simulink model "rev0BB"  (R2017b)
settings: Solver=FixedStepDiscrete  StartTime=0  StopTime=(((preLen+100+dataLenSymbols)*1+pad_first*3)*basePer)  RelTol=1e-3
values from neighbouring files (symbols this model uses):
  ack_stf_len_symbols = length(x_ACK_STF)    [rev0BB_setup.m]
  agc_delay_lag = 32    [rev0BB_setup.m]
  agc_detector_coef = ones(1,agc_detector_taps)./agc_detector_taps    [rev0BB_setup.m]
  agc_on = true    [rev0BB_startup.m]
  agc_sat_low = -agcSaturation    (= -12)    [rev0BB_setup.m]
  agc_sat_up = agcSaturation    (= 12)    [rev0BB_setup.m]
  agcDesired = 0    [rev0BB_setup.m]
  agcExpDomain = agcSaturation    (= 12)    [rev0BB_setup.m]
  agcExpResolution = 2^-5    (= 0.03125)    [rev0BB_setup.m]
  agcPwrAvgNum = 128    [rev0BB_setup.m]
  agcSaturation = 12    [rev0BB_setup.m]
  agcSettleThresh = 0.65    [rev0BB_setup.m]
  agcStep = 2^-8    (= 0.00390625)    [rev0BB_setup.m]
  atanDomain = 5    [rev0BB_setup.m]
  atanDomainTiming = 256    [rev0BB_setup.m]
  atanResolution = 2^-9    (= 0.001953125)    [rev0BB_setup.m]
  atanResolutionTiming = 2^-5    (= 0.03125)    [rev0BB_setup.m]
  averaging_num = ones(1, averaging_samples)    [rev0BB_setup.m]
  averaging_samples = 128    [rev0BB_setup.m]
  awgnSeed = abs(dBSnrRange(dBSnrInd)*1000+trial+10000000)    [plotBer.m]    (also in rev0BB_startup.m = 67)
  basePer = 1/baseFreq    (= 5e-08)    [rev0BB_setup.m]
  bitsPerSymbolHeader = log2(radixHeader)    [rev0BB_setup.m]
  bitsPerSymbolMax = log2(radixMax)    [rev0BB_setup.m]
  cal_sig_i_mult = 1.0    (= 1)    [rev0BB_startup.m]
  cal_sig_i_offset = 0.0    (= 0)    [rev0BB_startup.m]
  cal_sig_q_mult = 1.0    (= 1)    [rev0BB_startup.m]
  cal_sig_q_offset = 0.0    (= 0)    [rev0BB_startup.m]
  cefEarlyWarning = 256    [rev0BB_setup.m]
  cefLen = length(x_CEF)    [rev0BB_setup.m]
  channelFIR = zeros(1, round(maxSampleDelay)+1)    [rev0BB_startup.m]
  coarseCFOAdaptDelay = 1    [rev0BB_setup.m]
  cr_i = 0.020    (= 0.02)    [rev0BB_setup.m]
  cr_i_preamp = 2^-9    (= 0.001953125)    [rev0BB_setup.m]
  cr_int1_sat_low = -cr_integrator1_saturation    (= -0.6)    [rev0BB_setup.m]
  cr_int1_sat_up = cr_integrator1_saturation    (= 0.6)    [rev0BB_setup.m]
  cr_integrator1_decay = 1    [rev0BB_setup.m]
  cr_integrator1_saturation = 0.6    [rev0BB_setup.m]
  cr_mult_pipeline = 0    [rev0BB_setup.m]
  cr_p = 0.015    [rev0BB_setup.m]
  cr_sat2_low = -cr_saturation2    (= -0.6)    [rev0BB_setup.m]
  cr_sat2_up = cr_saturation2    (= 0.6)    [rev0BB_setup.m]
  cr_smooth_num = (1/cr_smooth_samples).*ones(1, cr_smooth_samples)    [rev0BB_setup.m]
  D_128 = [ 1,  8,  2,  4, 16, 32, 64]    [golay.m]    (also in rev0BB_setup.m)
  D_32 = [ 1,  4,  8,  2, 16]    [golay.m]    (also in rev0BB_setup.m)
  dataLenSymbols = header_len_bytes*8/bitsPerSymbolHeader + frame_len_bytes*8/bitsPerSymbol    [rev0BB_setup.m]
  default_channel = 3    [rev0BB_setup.m]
  dmm_coefs = ones(1,dmm_samples)./dmm_samples    [rev0BB_setup.m]
  dst_field_len = 8    [rev0BB_setup.m]
  expDomain = 3.3    [rev0BB_setup.m]
  expResolution = 2^-5    (= 0.03125)    [rev0BB_setup.m]
  expTol = .1    (= 0.1)    [rev0BB_setup.m]
  flush_delay = regular_pipeline*2+mult_pipeline+4    (= 4)    [rev0BB_setup.m]
  frac_lut_domain = 256    [rev0BB_setup.m]
  frac_lut_domain_cr = 64    [rev0BB_setup.m]
  frac_lut_range_max = 512    [rev0BB_setup.m]
  frac_lut_range_max_coarse_cfo = 127    [rev0BB_setup.m]
  frac_lut_range_max_cr = 127    [rev0BB_setup.m]
  frac_lut_range_min = -frac_lut_range_max    (= -512)    [rev0BB_setup.m]
  frac_lut_range_min_coarse_cfo = -frac_lut_range_max_coarse_cfo    (= -127)    [rev0BB_setup.m]
  frac_lut_range_min_cr = -frac_lut_range_max_cr    (= -127)    [rev0BB_setup.m]
  frac_lut_table_breaks = -frac_lut_domain:frac_lut_res:(frac_lut_domain-1)    [rev0BB_setup.m]
  frac_lut_table_breaks_coarse_cfo = -frac_lut_domain_coarse_cfo:frac_lut_res_coarse_cfo:(frac_lut_domain_coarse_cfo-1)    [rev0BB_setup.m]
  frac_lut_table_breaks_cr = -frac_lut_domain_cr:frac_lut_res_cr:(frac_lut_domain_cr-1)    [rev0BB_setup.m]
  frac_lut_table_data = 1./frac_lut_table_breaks    [rev0BB_setup.m]
  frac_lut_table_data_coarse_cfo = 1./frac_lut_table_breaks_coarse_cfo    [rev0BB_setup.m]
  frac_lut_table_data_cr = 1./frac_lut_table_breaks_cr    [rev0BB_setup.m]
  freeze_en_agc = true    [rev0BB_startup.m]
  freeze_en_cr_int1 = false    [rev0BB_startup.m]
  freeze_en_cr_int2 = false    [rev0BB_startup.m]
  freeze_en_cr_phase = false    [rev0BB_startup.m]
  freeze_en_tr_int1 = false    [rev0BB_startup.m]
  freeze_en_tr_int2 = false    [rev0BB_startup.m]
  freeze_en_tr_phase = false    [rev0BB_startup.m]
  freeze_on_cef_done = true    [rev0BB_startup.m]
  freeze_on_stf_done = false    [rev0BB_startup.m]
  freeze_on_valid = true    [rev0BB_startup.m]
  golay_type = 32    [rev0BB_setup.m]
  guardInt = int16(4)    [rev0BB_setup.m]
  guardTol = int16(5)    [rev0BB_setup.m]
  header_len_bytes = 8    [rev0BB_setup.m]
  lineWidth = 60    [rev0BB_setup.m]
  lmsEqDepth = 38    [rev0BB_setup.m]
  lmsStep_init = 0.006    [rev0BB_setup.m]
  lmsStep_meta = (lmsStep_final - lmsStep_init)/cefLen    [rev0BB_setup.m]
  lnDomain = 16    [rev0BB_setup.m]
  lnResolution = 2^-5    (= 0.03125)    [rev0BB_setup.m]
  local_node_id = 2    [rev0BB_startup.m]
  maxMsgSize = length(xSpectrum_PRE)+dataLenSymbols+300    [rev0BB_setup.m]
  minSTFPeaks = 3    [rev0BB_setup.m]
  mod_scheme_len_bytes = 1    [rev0BB_setup.m]
  modBPS = [1, 2, 4]    [rev0BB_setup.m]
  modKeys = [0, 1, 2]    [rev0BB_setup.m]
  mult_pipeline = 0    [rev0BB_setup.m]
  overSampleFreq = 80e6    (= 80000000)    [rev0BB_setup.m]
  overSamplePer = 1/overSampleFreq    (= 1.25e-08)    [rev0BB_setup.m]
  pad_first = 1000    [createTestVectors.m]
  post_cr_i_offset = 0    [rev0BB_startup.m]
  post_cr_q_offset = 0    [rev0BB_startup.m]
  preambleSequentialDetect = 2    [rev0BB_setup.m]
  preLen = length(x_PRE)    [rev0BB_setup.m]
  qam16_demod_scale_factor = qam16_hdl_distance/qam16_power_normalized_distance    [rev0BB_setup.m]
  rcRxFilt = [0.000303163120401141 -0.00118915940834234 -0.00187387637177 -0.00124167532697737 0.00029186889076529 0.00164526160586517 0.00182432050803312 0.000652133621739543 -0.00105668254004908 -0.00204011570659167 -0.00150058088768918 0.00026138356356816 0.0019831869994874 0.00231075800085521 0.000821993419120097 -0.00154687337975486 -0.00305430783933469 -0.00238186490079127 0.000301216962040692 0.00325307 ...(+2001 chars)    [rev0BB_setup.m]
  rcTxFilt = [0.000303163120401141 -0.00118915940834234 -0.00187387637177 -0.00124167532697737 0.00029186889076529 0.00164526160586517 0.00182432050803312 0.000652133621739543 -0.00105668254004908 -0.00204011570659167 -0.00150058088768918 0.00026138356356816 0.0019831869994874 0.00231075800085521 0.000821993419120097 -0.00154687337975486 -0.00305430783933469 -0.00238186490079127 0.000301216962040692 0.00325307 ...(+2001 chars)    [rev0BB_setup.m]
  regular_pipeline = 0    [rev0BB_setup.m]
  rx_gain = 1    [rev0BB_setup.m]
  rx_gain_i = 1    [rev0BB_setup.m]
  rx_gain_q = 1    [rev0BB_setup.m]
  rx_impare_i_offset = 0    [rev0BB_startup.m]
  rx_impare_i_scale = 1    [rev0BB_startup.m]
  rx_impare_q_offset = 0    [rev0BB_startup.m]
  rx_impare_q_scale = 1    [rev0BB_startup.m]
  rx_offset_correction_i = 0    [rev0BB_startup.m]
  rx_offset_correction_q = 0    [rev0BB_startup.m]
  sin_source_amp = 1    [rev0BB_setup.m]
  sin_source_freq = 250e6/16    (= 15625000)    [rev0BB_setup.m]
  slowPer = overSamplePer*slowSample    (= 2.5e-08)    [rev0BB_setup.m]
  std_pkt_type = 0    [rev0BB_setup.m]
  stfLen = length(x_STF)    [rev0BB_setup.m]
  testMsg = cat(1, xCTRL_PRE_adj, header, payload)    [plotBer.m]
  timing_i = 0.25    [rev0BB_setup.m]
  ... (+25 more)
undefined symbols (not defined in the file or in its folder): cr_integrator2_saturation, doppler, i, magnitude, useFadingChannel
libraries: helperLib x128, simulink x90, golayLib x34, dspsigops x32, commfilt2 x27, commdigbbndpm3 x8, hdlsllib x6, dsparch4 x4, commdigbbndam3 x4, commchan3 x2, commrflib2 x2, commcrc2 x2
(part 9 of 10)

== system rev0BB/receiver/slow_rx_baseband_outer/slow_rx_baseband_enabled/slow_rx_baseband/FineCarrierRecovery/Est_Phase/atan2 ==
  note: 4 delays
  note: Special case for undefined ouput of atan2.
      | To produce an unbiased ouput, this should be 0.
  imag_y : Inport
  real_x : Inport  Port=2
  Add : Sum
  Compare To Constant1 : simulink/Logic and Bit Operations/Compare To Constant  relop=>=  const=0  OutDataTypeStr=boolean
  Compare To Constant2 : simulink/Logic and Bit Operations/Compare To Constant  relop=>=  const=0  OutDataTypeStr=boolean
  Compare To Constant3 : simulink/Logic and Bit Operations/Compare To Constant  relop===  const=0  OutDataTypeStr=boolean
  Compare To Constant4 : simulink/Logic and Bit Operations/Compare To Constant  relop===  const=0  OutDataTypeStr=boolean
  Constant : Constant  Value=pi  OutDataTypeStr=Inherit: Inherit via back propagation  SampleTime=-1
  Constant2 : Constant  Value=0  OutDataTypeStr=Inherit: Inherit via back propagation  SampleTime=-1
  Constant3 : Constant  Value=-pi/2  OutDataTypeStr=Inherit: Inherit via back propagation  SampleTime=-1
  Constant4 : Constant  Value=pi/2  OutDataTypeStr=Inherit: Inherit via back propagation  SampleTime=-1
  Logical Operator : Logic  AllPortsSameDT=off  OutDataTypeStr=boolean
  Logical Operator1 : Logic  AllPortsSameDT=off  OutDataTypeStr=boolean
  Sub : Sum  Inputs=+-
  Switch{1,3..5,8} (5 alike) : Switch  Criteria=u2 ~= 0  OutDataTypeStr=Inherit: Inherit via back propagation
  bound_atan : Subsystem  AncestorBlock=helperLib/bound_atan
  inv : Subsystem
  mult_delay_match : Delay  DelayLength=cr_mult_pipeline*2+regular_pipeline*2
  pipeline_delay{,1..3} (4 alike) : Delay  DelayLength=regular_pipeline
  pipeline_delay_match{,1..4} (5 alike) : Delay  DelayLength=cr_mult_pipeline*5+regular_pipeline*7
  pipelined_mult : helperLib/pipelined_mult  d=cr_mult_pipeline
  Out1 : Outport
  wires:
  pipeline_delay1/1 -> bound_atan/1(In1)
  pipeline_delay_match/1 -> Switch1/2
  pipeline_delay_match1/1 -> Switch8/2
  imag_y/1 -> Compare To Constant4/1, Logical Operator1/1, Compare To Constant2/1, mult_delay_match/1
  Sub/1 -> Switch1/3
  Constant/1 -> Sub/2, Add/2
  Add/1 -> Switch1/1
  Switch1/1 -> Switch8/3
  Compare To Constant2/1 -> pipeline_delay_match/1
  Compare To Constant1/1 -> pipeline_delay_match1/1
  pipeline_delay/1 -> Sub/1, Add/1, Switch8/1
  mult_delay_match/1 -> pipeline_delay2/1
  bound_atan/1(Out1) -> pipeline_delay/1
  pipelined_mult/1 -> pipeline_delay1/1
  pipeline_delay2/1 -> pipelined_mult/1
  pipeline_delay3/1 -> pipelined_mult/2
  Compare To Constant4/1 -> Logical Operator/1
  Logical Operator/1 -> pipeline_delay_match2/1
  pipeline_delay_match2/1 -> Switch3/2
  real_x/1 -> inv/1(In), Compare To Constant3/1, Compare To Constant1/1
  inv/1(Out) -> pipeline_delay3/1
  Switch8/1 -> Switch4/3
  Switch4/1 -> Switch5/3
  Constant3/1 -> Switch4/1
  Constant4/1 -> Switch5/1
  Switch5/1 -> Switch3/3
  Constant2/1 -> Switch3/1
  Switch3/1 -> Out1/1
  Compare To Constant3/1 -> Logical Operator1/2, pipeline_delay_match4/1, Logical Operator/2
  Logical Operator1/1 -> pipeline_delay_match3/1
  pipeline_delay_match3/1 -> Switch5/2
  pipeline_delay_match4/1 -> Switch4/2

== system rev0BB/receiver/slow_rx_baseband_outer/slow_rx_baseband_enabled/slow_rx_baseband/FineCarrierRecovery/Est_Phase/complex_mult_pipelined1 ==
  In1 : Inport
  In2 : Inport  Port=2
  Add1 : Sum  OutDataTypeStr=Inherit: Same as first input
  Add2 : Sum  OutDataTypeStr=Inherit: Same as first input
  Complex to Real-Imag3 : ComplexToRealImag
  Complex to Real-Imag4 : ComplexToRealImag
  Real-Imag to Complex2 : RealImagToComplex
  mult_delay_match3 : Delay  DelayLength=cr_mult_pipeline
  mult_delay_match4 : Delay  DelayLength=cr_mult_pipeline
  mult_delay_match5 : Delay  DelayLength=cr_mult_pipeline
  pipeline_delay{1..3,6} (4 alike) : Delay  DelayLength=regular_pipeline
  pipelined_gain : helperLib/pipelined_gain  g=-1  d=cr_mult_pipeline
  pipelined_mult{,1..3} (4 alike) : helperLib/pipelined_mult  d=cr_mult_pipeline
  Out1 : Outport
  wires:
  pipelined_gain/1 -> Add1/2
  pipelined_mult3/1 -> mult_delay_match5/1
  pipelined_mult2/1 -> mult_delay_match4/1
  pipelined_mult1/1 -> pipelined_gain/1
  pipelined_mult/1 -> mult_delay_match3/1
  Complex to Real-Imag4/1 -> pipelined_mult/2, pipelined_mult3/2
  Complex to Real-Imag3/2 -> pipelined_mult1/1, pipelined_mult3/1
  Complex to Real-Imag4/2 -> pipelined_mult2/2, pipelined_mult1/2
  Complex to Real-Imag3/1 -> pipelined_mult2/1, pipelined_mult/1
  pipeline_delay3/1 -> Complex to Real-Imag4/1
  pipeline_delay2/1 -> Complex to Real-Imag3/1
  Add2/1 -> pipeline_delay6/1
  Add1/1 -> pipeline_delay1/1
  In1/1 -> pipeline_delay2/1
  mult_delay_match5/1 -> Add2/2
  pipeline_delay1/1 -> Real-Imag to Complex2/1
  In2/1 -> pipeline_delay3/1
  pipeline_delay6/1 -> Real-Imag to Complex2/2
  Real-Imag to Complex2/1 -> Out1/1
  mult_delay_match3/1 -> Add1/1
  mult_delay_match4/1 -> Add2/1

== system rev0BB/receiver/slow_rx_baseband_outer/slow_rx_baseband_enabled/slow_rx_baseband/FineCarrierRecovery/Est_Phase/find_nearest ==
  In1 : Inport
  ModMode : Inport  Port=2
  BPSK Demodulator Baseband : commdigbbndpm3/BPSK Demodulator Baseband  DecType=Hard decision  VarSource=Dialog  Variance=1  Ph=0  outDtype=boolean  derotateFactorWordLen=16  derotateFactorDataTypeStr=Inherit: Same word length as input  derotateFactorLastDataTypeStr=Inherit: Same word length as input
  BPSK Modulator Baseband : commdigbbndpm3/BPSK Modulator Baseband  Ph=0  outDtype=single  outWordLen=25  outUDDataType=sfix(16)  outFracLenMode=User-defined  outFracLen=17  outDataTypeStr=single  outLastDataTypeStr=single
  Gain : Gain  Gain=qam16_demod_scale_factor
  Multiport Switch : MultiPortSwitch
  QAM16 Scale Diagram : ConstellationDiagram  Commented=on
  QPSK Demodulator Baseband : commdigbbndpm3/QPSK Demodulator Baseband  OutType=Integer  DecType=Hard decision  VarSource=Dialog  Variance=1  Dec=Gray  Ph=pi/4  outDtype1=Inherit via internal rule  outDtype2=uint8  derotateFactorWordLen=16  derotateFactorDataTypeStr=Inherit: Same word length as input  derotateFactorLastDataTypeStr=Inherit: Same word length as input
  QPSK Modulator Baseband : commdigbbndpm3/QPSK Modulator Baseband  InType=Integer  Enc=Gray  Ph=pi/4  outDtype=single  outWordLen=25  outUDDataType=sfix(16)  outFracLenMode=User-defined  outFracLen=17  outDataTypeStr=single  outLastDataTypeStr=single
  Rectangular QAM Demodulator Baseband1 : commdigbbndam3/Rectangular QAM Demodulator Baseband  M=16  OutType=Integer  DecType=Hard decision  VarSource=Dialog  Variance=1  Dec=Gray  Mapping=[0:15]  PowType=Min. distance between symbols  MinDist=qam16_hdl_distance  AvgPow=1  PeakPow=1  Ph=0  outDtype1=Inherit via internal rule  outDtype2=uint8  derotateFactorWordLen=16  derotateFactorDataTypeStr=Inherit: Same word length as input  derotateFactorLastDataTypeStr=Inherit: Same word length as input  denormFactorWordLen=16  denormFactorDataTypeStr=Inherit: Same word length as input  denormFactorLastDataTypeStr=Inherit: Same word length as input  prodOutWordLen=32  prodOutOverflowMode=Wrap  prodOutRoundingMode=Floor  prodOutOvFlMode=off  prodOutOvFlModeLastStrValue=off  sumWordLen=32
  Rectangular QAM Modulator Baseband : commdigbbndam3/Rectangular QAM Modulator Baseband  M=16  InType=Integer  Enc=Gray  Mapping=[0:15]  PowType=Average Power  MinDist=2  AvgPow=1  PeakPow=1  Ph=0  outDtype=single  outWordLen=25  outUDDataType=sfix(16)  outFracLenMode=User-defined  outFracLen=17  outDataTypeStr=single  outLastDataTypeStr=single
  Out1 : Outport
  wires:
  BPSK Demodulator Baseband/1 -> BPSK Modulator Baseband/1
  In1/1 -> Gain/1, QPSK Demodulator Baseband/1, BPSK Demodulator Baseband/1
  QPSK Demodulator Baseband/1 -> QPSK Modulator Baseband/1
  Multiport Switch/1 -> Out1/1
  BPSK Modulator Baseband/1 -> Multiport Switch/2
  QPSK Modulator Baseband/1 -> Multiport Switch/3
  Rectangular QAM Modulator Baseband/1 -> Multiport Switch/4
  ModMode/1 -> Multiport Switch/1
  Gain/1 -> QAM16 Scale Diagram/1, Rectangular QAM Demodulator Baseband1/1
  Rectangular QAM Demodulator Baseband1/1 -> Rectangular QAM Modulator Baseband/1

== system rev0BB/receiver/slow_rx_baseband_outer/slow_rx_baseband_enabled/slow_rx_baseband/FineCarrierRecovery/scale_and_loop/Loop Filter ==
  PhaseOffset : Inport
  cr_i_preamp : Inport  Port=2
  cr_p : Inport  Port=3
  cr_i : Inport  Port=4
  cr_integrator1_decay : Inport  Port=5
  cr_int1_sat_up : Inport  Port=6
  cr_int1_sat_low : Inport  Port=7
  cr_sat2_up : Inport  Port=8
  cr_sat2_low : Inport  Port=9
  int1_freeze : Inport  Port=10  OutDataTypeStr=boolean
  reset : Inport  Port=11
  Add1 : Sum  OutDataTypeStr=Inherit: Same as first input
  Add2 : Sum  OutDataTypeStr=Inherit: Same as first input
  Constant : Constant  Value=0  OutDataTypeStr=Inherit: Inherit via back propagation  SampleTime=-1
  Constant1 : Constant  Value=0  OutDataTypeStr=Inherit: Inherit via back propagation  SampleTime=-1
  Data Type Duplicate{1..3,5} (4 alike) : DataTypeDuplicate
  Delay1 : Delay  DelayLength=1  InitialCondition=0
  Discrete FIR Filter : DiscreteFir  FilterStructure=Direct form transposed  Coefficients=cr_smooth_num  OutDataTypeStr=Inherit: Same as input
  Switch1 : Switch  Criteria=u2 > Threshold
  Switch2 : Switch  Criteria=u2 > Threshold
  Switch3 : Switch  Criteria=u2 > Threshold
  cr_components : Scope  NumInputPorts=2
  pipeline_delay{3..8} (6 alike) : Delay  DelayLength=regular_pipeline
  pipelined_mult{,1..2,4} (4 alike) : helperLib/pipelined_mult  d=cr_mult_pipeline
  sat : Subsystem
  sat2 : Subsystem
  Out : Outport
  wires:
  Add1/1 -> sat/1(In1)
  Switch2/1 -> Add2/1
  pipeline_delay5/1 -> Add1/1
  PhaseOffset/1 -> pipeline_delay8/1
  sat/1(Out1) -> pipelined_mult2/1, Data Type Duplicate5/1, pipelined_mult4/1, Data Type Duplicate3/1
  cr_p/1 -> pipelined_mult/2, Data Type Duplicate2/2
  Discrete FIR Filter/1 -> Data Type Duplicate2/1, pipelined_mult/1, Data Type Duplicate1/1, pipelined_mult1/1
  cr_i_preamp/1 -> pipelined_mult1/2, Data Type Duplicate1/2
  pipelined_mult1/1 -> pipeline_delay5/1
  cr_i/1 -> pipelined_mult2/2, Data Type Duplicate3/2
  pipelined_mult2/1 -> pipeline_delay4/1
  cr_integrator1_decay/1 -> Data Type Duplicate5/2, pipelined_mult4/2
  pipelined_mult/1 -> pipeline_delay3/1
  cr_int1_sat_up/1 -> sat/2(limit_up)
  cr_int1_sat_low/1 -> sat/3(limit_low)
  cr_sat2_up/1 -> sat2/2(limit_up)
  cr_sat2_low/1 -> sat2/3(limit_low)
  Delay1/1 -> Switch1/1
  int1_freeze/1 -> Switch2/2, Switch1/2
  Switch1/1 -> Delay1/1, Add2/2
  pipeline_delay4/1 -> cr_components/2, Switch1/3
  pipeline_delay3/1 -> cr_components/1, Switch2/3
  Constant/1 -> Switch2/1
  pipeline_delay8/1 -> Discrete FIR Filter/1
  pipeline_delay7/1 -> sat2/1(In1)
  sat2/1(Out1) -> pipeline_delay6/1
  pipeline_delay6/1 -> Out/1
  Add2/1 -> pipeline_delay7/1
  pipelined_mult4/1 -> Switch3/3
  Switch3/1 -> Add1/2
  Constant1/1 -> Switch3/1
  reset/1 -> Switch3/2

== system rev0BB/receiver/fast_rx_baseband/Timing Recovery/nda_4x_time_err_enable/phase_est/timing_rec_sym_rate_enb/atan2/bound_atan ==
  note: Bound Protection
  In1 : Inport
  Compare To Constant1 : simulink/Logic and Bit Operations/Compare To Constant  relop=>=  const=atanDomainTiming-1  OutDataTypeStr=boolean
  Compare To Constant4 : simulink/Logic and Bit Operations/Compare To Constant  relop=<=  const=-atanDomainTiming  OutDataTypeStr=boolean
  Constant11 : Constant  Value=0  OutDataTypeStr=Inherit: Inherit via back propagation  SampleTime=-1
  Constant3 : Constant  Value=pi/2  OutDataTypeStr=Inherit: Inherit via back propagation  SampleTime=-1
  Constant4 : Constant  Value=-pi/2  OutDataTypeStr=Inherit: Inherit via back propagation  SampleTime=-1
  Data Type Duplicate : DataTypeDuplicate
  Data Type Duplicate1 : DataTypeDuplicate
  Data Type Duplicate2 : DataTypeDuplicate
  Data Type Conversion : DataTypeConversion  OutDataTypeStr=single
  Logical Operator : Logic  Operator=OR  AllPortsSameDT=off  OutDataTypeStr=boolean
  Switch2 : Switch  Criteria=u2 ~= 0  OutDataTypeStr=Inherit: Inherit via back propagation
  Switch3 : Switch  Criteria=u2 ~= 0  OutDataTypeStr=Inherit: Inherit via back propagation
  Switch8 : Switch  Criteria=u2 ~= 0  OutDataTypeStr=Inherit: Inherit via back propagation
  atan Lookup Table : Lookup_n-D  NumberOfTableDimensions=1  BreakpointsForDimension1=[-atanDomainTiming:atanResolutionTiming:(atanDomainTiming-1)]  IndexSearchMethod=Evenly spaced points  Table=atan([-atanDomainTiming:atanResolutionTiming:(atanDomainTiming-1)])  InterpMethod=Flat  DiagnosticForOutOfRangeInput=Error  RemoveProtectionInput=on  InternalRulePriority=Speed  OutDataTypeStr=Inherit: Inherit via back propagation  RndMeth=Simplest  InputSameDT=on
  mult_delay : Delay  DelayLength=wide_mult_pipeline
  mult_delay_match : Delay  DelayLength=wide_mult_pipeline
  mult_delay_match1 : Delay  DelayLength=wide_mult_pipeline
  pipeline_delay1 : Delay  DelayLength=regular_pipeline*3
  pipeline_delay2 : Delay  DelayLength=regular_pipeline
  pipeline_delay3 : Delay  DelayLength=regular_pipeline
  pipeline_delay_match : Delay  DelayLength=regular_pipeline*3
  pipeline_delay_match1 : Delay  DelayLength=regular_pipeline*3
  Out1 : Outport
  wires:
  mult_delay/1 -> Data Type Duplicate2/1, Switch2/3
  pipeline_delay1/1 -> atan Lookup Table/1
  mult_delay_match1/1 -> Switch3/2
  mult_delay_match/1 -> Switch2/2
  pipeline_delay_match1/1 -> mult_delay_match1/1
  pipeline_delay_match/1 -> mult_delay_match/1
  atan Lookup Table/1 -> Data Type Duplicate/2, mult_delay/1
  Switch8/1 -> Data Type Conversion/1
  Constant11/1 -> Switch8/1
  Logical Operator/1 -> Switch8/2
  In1/1 -> pipeline_delay2/1
  Switch3/1 -> pipeline_delay3/1
  Constant4/1 -> Switch3/1
  Switch2/1 -> Data Type Duplicate1/1, Switch3/3
  Constant3/1 -> Switch2/1
  Compare To Constant4/1 -> pipeline_delay_match1/1, Logical Operator/2
  Compare To Constant1/1 -> pipeline_delay_match/1, Logical Operator/1
  pipeline_delay2/1 -> Data Type Duplicate/1, Compare To Constant4/1, Compare To Constant1/1, Switch8/3
  pipeline_delay3/1 -> Data Type Duplicate2/2, Data Type Duplicate1/2, Out1/1
  Data Type Conversion/1 -> pipeline_delay1/1

== system rev0BB/receiver/fast_rx_baseband/Timing Recovery/nda_4x_time_err_enable/phase_est/timing_rec_sym_rate_enb/atan2/inv ==
  note: Bound Protection
  In : Inport
  Compare To Constant1 : simulink/Logic and Bit Operations/Compare To Constant  relop=>=  const=frac_lut_domain-1  OutDataTypeStr=boolean
  Compare To Constant4 : simulink/Logic and Bit Operations/Compare To Constant  relop=<=  const=-frac_lut_domain  OutDataTypeStr=boolean
  Constant11 : Constant  Value=0  OutDataTypeStr=Inherit: Inherit via back propagation  SampleTime=-1
  Constant3 : Constant  Value=frac_lut_range_max  OutDataTypeStr=Inherit: Inherit via back propagation  SampleTime=-1
  Constant4 : Constant  Value=frac_lut_range_min  OutDataTypeStr=Inherit: Inherit via back propagation  SampleTime=-1
  Data Type Duplicate : DataTypeDuplicate
  Data Type Duplicate1 : DataTypeDuplicate
  Data Type Duplicate2 : DataTypeDuplicate
  Data Type Conversion : DataTypeConversion  OutDataTypeStr=single
  Logical Operator : Logic  Operator=OR  AllPortsSameDT=off  OutDataTypeStr=boolean
  Switch2 : Switch  Criteria=u2 ~= 0  OutDataTypeStr=Inherit: Inherit via back propagation
  Switch3 : Switch  Criteria=u2 ~= 0  OutDataTypeStr=Inherit: Inherit via back propagation
  Switch8 : Switch  Criteria=u2 ~= 0  OutDataTypeStr=Inherit: Inherit via back propagation
  exp Lookup Table : Lookup_n-D  NumberOfTableDimensions=1  BreakpointsForDimension1=frac_lut_table_breaks  IndexSearchMethod=Evenly spaced points  Table=frac_lut_table_data  InterpMethod=Flat  DiagnosticForOutOfRangeInput=Error  RemoveProtectionInput=on  InternalRulePriority=Speed  OutDataTypeStr=Inherit: Inherit via back propagation  RndMeth=Simplest  InputSameDT=on
  mult_delay : Delay  DelayLength=wide_mult_pipeline
  mult_delay_match : Delay  DelayLength=wide_mult_pipeline
  mult_delay_match1 : Delay  DelayLength=wide_mult_pipeline
  pipeline_delay1 : Delay  DelayLength=regular_pipeline
  pipeline_delay2 : Delay  DelayLength=regular_pipeline*3  InitialCondition=1
  pipeline_delay_match : Delay  DelayLength=regular_pipeline*4
  pipeline_delay_match1 : Delay  DelayLength=regular_pipeline*4
  Out : Outport
  wires:
  pipeline_delay2/1 -> Data Type Duplicate2/1, Switch2/3
  mult_delay/1 -> exp Lookup Table/1
  mult_delay_match1/1 -> Switch3/2
  mult_delay_match/1 -> Switch2/2
  pipeline_delay_match1/1 -> mult_delay_match1/1
  pipeline_delay_match/1 -> mult_delay_match/1
  exp Lookup Table/1 -> Data Type Duplicate/2, pipeline_delay2/1
  Switch8/1 -> Data Type Conversion/1
  Constant11/1 -> Switch8/1
  Logical Operator/1 -> Switch8/2
  Switch3/1 -> Data Type Duplicate2/2, Data Type Duplicate1/2, Out/1
  Constant4/1 -> Switch3/1
  Switch2/1 -> Data Type Duplicate1/1, Switch3/3
  Constant3/1 -> Switch2/1
  Compare To Constant4/1 -> pipeline_delay_match1/1, Logical Operator/2
  Compare To Constant1/1 -> pipeline_delay_match/1, Logical Operator/1
  In/1 -> Data Type Duplicate/1, Compare To Constant4/1, Compare To Constant1/1, Switch8/3
  Data Type Conversion/1 -> pipeline_delay1/1
  pipeline_delay1/1 -> mult_delay/1

== system rev0BB/receiver/slow_rx_baseband_outer/slow_rx_baseband_enabled/slow_rx_baseband/FineCarrierRecovery/Est_Phase/atan2/bound_atan ==
  note: Bound Protection
  In1 : Inport
  Compare To Constant1 : simulink/Logic and Bit Operations/Compare To Constant  relop=>=  const=atanDomain  OutDataTypeStr=boolean
  Compare To Constant4 : simulink/Logic and Bit Operations/Compare To Constant  relop=<=  const=-atanDomain  OutDataTypeStr=boolean
  Constant11 : Constant  Value=0  OutDataTypeStr=Inherit: Inherit via back propagation  SampleTime=-1
  Constant3 : Constant  Value=pi/2  OutDataTypeStr=Inherit: Inherit via back propagation  SampleTime=-1
  Constant4 : Constant  Value=-pi/2  OutDataTypeStr=Inherit: Inherit via back propagation  SampleTime=-1
  Data Type Duplicate : DataTypeDuplicate
  Data Type Duplicate1 : DataTypeDuplicate
  Data Type Duplicate2 : DataTypeDuplicate
  Data Type Conversion : DataTypeConversion  OutDataTypeStr=single
  Logical Operator : Logic  Operator=OR  AllPortsSameDT=off  OutDataTypeStr=boolean
  Switch2 : Switch  Criteria=u2 ~= 0  OutDataTypeStr=Inherit: Inherit via back propagation
  Switch3 : Switch  Criteria=u2 ~= 0  OutDataTypeStr=Inherit: Inherit via back propagation
  Switch8 : Switch  Criteria=u2 ~= 0  OutDataTypeStr=Inherit: Inherit via back propagation
  atan Lookup Table : Lookup_n-D  NumberOfTableDimensions=1  BreakpointsForDimension1=[-atanDomain:atanResolution:atanDomain]  IndexSearchMethod=Evenly spaced points  Table=atan([-atanDomain:atanResolution:atanDomain])  InterpMethod=Flat  DiagnosticForOutOfRangeInput=Error  RemoveProtectionInput=on  InternalRulePriority=Speed  OutDataTypeStr=Inherit: Inherit via back propagation  RndMeth=Simplest  InputSameDT=on
  mult_delay : Delay  DelayLength=cr_mult_pipeline
  mult_delay_match : Delay  DelayLength=cr_mult_pipeline
  mult_delay_match1 : Delay  DelayLength=cr_mult_pipeline
  pipeline_delay1 : Delay  DelayLength=regular_pipeline*2
  pipeline_delay2 : Delay  DelayLength=regular_pipeline
  pipeline_delay_match : Delay  DelayLength=regular_pipeline*3
  pipeline_delay_match1 : Delay  DelayLength=regular_pipeline*3
  Out1 : Outport
  wires:
  pipeline_delay2/1 -> Data Type Duplicate2/1, Switch2/3
  mult_delay/1 -> atan Lookup Table/1
  pipeline_delay1/1 -> mult_delay/1
  mult_delay_match1/1 -> Switch3/2
  mult_delay_match/1 -> Switch2/2
  pipeline_delay_match1/1 -> mult_delay_match1/1
  pipeline_delay_match/1 -> mult_delay_match/1
  atan Lookup Table/1 -> Data Type Duplicate/2, pipeline_delay2/1
  Switch8/1 -> Data Type Conversion/1
  Constant11/1 -> Switch8/1
  Logical Operator/1 -> Switch8/2
  In1/1 -> Data Type Duplicate/1, Compare To Constant4/1, Compare To Constant1/1, Switch8/3
  Switch3/1 -> Data Type Duplicate2/2, Data Type Duplicate1/2, Out1/1
  Constant4/1 -> Switch3/1
  Switch2/1 -> Data Type Duplicate1/1, Switch3/3
  Constant3/1 -> Switch2/1
  Compare To Constant4/1 -> pipeline_delay_match1/1, Logical Operator/2
  Compare To Constant1/1 -> pipeline_delay_match/1, Logical Operator/1
  Data Type Conversion/1 -> pipeline_delay1/1

== system rev0BB/receiver/slow_rx_baseband_outer/slow_rx_baseband_enabled/slow_rx_baseband/FineCarrierRecovery/Est_Phase/atan2/inv ==
  note: Bound Protection
  In : Inport
  Compare To Constant1 : simulink/Logic and Bit Operations/Compare To Constant  relop=>=  const=frac_lut_domain_cr-1  OutDataTypeStr=boolean
  Compare To Constant4 : simulink/Logic and Bit Operations/Compare To Constant  relop=<=  const=-frac_lut_domain_cr  OutDataTypeStr=boolean
  Constant11 : Constant  Value=0  OutDataTypeStr=Inherit: Inherit via back propagation  SampleTime=-1
  Constant3 : Constant  Value=frac_lut_range_max_cr  OutDataTypeStr=Inherit: Inherit via back propagation  SampleTime=-1
  Constant4 : Constant  Value=frac_lut_range_min_cr  OutDataTypeStr=Inherit: Inherit via back propagation  SampleTime=-1
  Data Type Duplicate : DataTypeDuplicate
  Data Type Duplicate1 : DataTypeDuplicate
  Data Type Duplicate2 : DataTypeDuplicate
  Data Type Conversion : DataTypeConversion  OutDataTypeStr=single
  Logical Operator : Logic  Operator=OR  AllPortsSameDT=off  OutDataTypeStr=boolean
  Switch2 : Switch  Criteria=u2 ~= 0  OutDataTypeStr=Inherit: Inherit via back propagation
  Switch3 : Switch  Criteria=u2 ~= 0  OutDataTypeStr=Inherit: Inherit via back propagation
  Switch8 : Switch  Criteria=u2 ~= 0  OutDataTypeStr=Inherit: Inherit via back propagation
  exp Lookup Table : Lookup_n-D  NumberOfTableDimensions=1  BreakpointsForDimension1=frac_lut_table_breaks_cr  IndexSearchMethod=Evenly spaced points  Table=frac_lut_table_data_cr  InterpMethod=Flat  DiagnosticForOutOfRangeInput=Error  RemoveProtectionInput=on  InternalRulePriority=Speed  OutDataTypeStr=Inherit: Inherit via back propagation  RndMeth=Simplest  InputSameDT=on
  mult_delay : Delay  DelayLength=cr_mult_pipeline*2
  mult_delay_match : Delay  DelayLength=cr_mult_pipeline*2
  mult_delay_match1 : Delay  DelayLength=cr_mult_pipeline*2
  pipeline_delay1 : Delay  DelayLength=regular_pipeline
  pipeline_delay2 : Delay  DelayLength=regular_pipeline  InitialCondition=1
  pipeline_delay_match : Delay  DelayLength=regular_pipeline*2
  pipeline_delay_match1 : Delay  DelayLength=regular_pipeline*2
  Out : Outport
  wires:
  pipeline_delay2/1 -> Data Type Duplicate2/1, Switch2/3
  mult_delay/1 -> exp Lookup Table/1
  pipeline_delay1/1 -> mult_delay/1
  mult_delay_match1/1 -> Switch3/2
  mult_delay_match/1 -> Switch2/2
  pipeline_delay_match1/1 -> mult_delay_match1/1
  pipeline_delay_match/1 -> mult_delay_match/1
  exp Lookup Table/1 -> Data Type Duplicate/2, pipeline_delay2/1
  Switch8/1 -> Data Type Conversion/1
  Constant11/1 -> Switch8/1
  Logical Operator/1 -> Switch8/2
  Switch3/1 -> Data Type Duplicate2/2, Data Type Duplicate1/2, Out/1
  Constant4/1 -> Switch3/1
  Switch2/1 -> Data Type Duplicate1/1, Switch3/3
  Constant3/1 -> Switch2/1
  Compare To Constant4/1 -> pipeline_delay_match1/1, Logical Operator/2
  Compare To Constant1/1 -> pipeline_delay_match/1, Logical Operator/1
  In/1 -> Data Type Duplicate/1, Compare To Constant4/1, Compare To Constant1/1, Switch8/3
  Data Type Conversion/1 -> pipeline_delay1/1

== system rev0BB/receiver/slow_rx_baseband_outer/slow_rx_baseband_enabled/slow_rx_baseband/FineCarrierRecovery/scale_and_loop/Loop Filter/sat ==
  In1 : Inport
  limit_up : Inport  Port=2
  limit_low : Inport  Port=3
  Saturation : Saturate  Commented=on  UpperLimit=cr_integrator1_saturation  LowerLimit=-cr_integrator1_saturation
  Saturation Dynamic : simulink/Discontinuities/Saturation Dynamic  OutMin=[]  OutMax=[]  OutDataTypeStr=Inherit: Same as second input  OutDataType=fixdt(1, 16)  OutScaling=2^-10  DoSatur=off
  pipeline_delay : Delay  DelayLength=regular_pipeline
  Out1 : Outport
  wires:
  In1/1 -> pipeline_delay/1
  pipeline_delay/1 -> Saturation Dynamic/2
  limit_up/1 -> Saturation Dynamic/1
  limit_low/1 -> Saturation Dynamic/3
  Saturation Dynamic/1 -> Out1/1

== system rev0BB/receiver/slow_rx_baseband_outer/slow_rx_baseband_enabled/slow_rx_baseband/FineCarrierRecovery/scale_and_loop/Loop Filter/sat2 ==
  In1 : Inport
  limit_up : Inport  Port=2
  limit_low : Inport  Port=3
  Saturation : Saturate  Commented=on  UpperLimit=cr_integrator2_saturation  LowerLimit=-cr_integrator2_saturation
  Saturation Dynamic : simulink/Discontinuities/Saturation Dynamic  OutMin=[]  OutMax=[]  OutDataTypeStr=Inherit: Same as second input  OutDataType=fixdt(1, 16)  OutScaling=2^-10  DoSatur=off
  pipeline_delay : Delay  DelayLength=regular_pipeline
  Out1 : Outport
  wires:
  In1/1 -> pipeline_delay/1
  limit_up/1 -> Saturation Dynamic/1
  limit_low/1 -> Saturation Dynamic/3
  pipeline_delay/1 -> Saturation Dynamic/2
  Saturation Dynamic/1 -> Out1/1

== stateflow chart rev0BB/receiver/slim_fast_rx/preamble_detect ==
  settings: executeAtInitialization=1
  state Lost
    entry:
    err = true;
    possible=false;
    periodCount = int32(0);
  state Reset
    entry:
    err=false;
    detected=false;
    possible=false;
    periodCount = int32(0);
    peakCount = int32(0);
  state WaitForNext
    entry:
    periodCount = periodCount + int32(1);
  state CalculateDiff
    entry:
    peakCount = peakCount + int32(1);
    periodCount = int32(1);
  state BufferFirst
    entry:
    periodCount = int32(1);
    possible=true;
  state SequentialDetected
    entry:
    detected=true;
  CalculateDiff -> Reset [order 1] : [rst == true]
  WaitForNext -> Reset [order 1] : [rst == true]
  WaitForNext -> Lost [order 2] : [periodCount > golay_type*4+4]
  Lost -> Reset
  CalculateDiff -> WaitForNext [order 3]
  BufferFirst -> Reset [order 1] : [rst == true]
  Reset -> BufferFirst : [peak == true]
  WaitForNext -> CalculateDiff [order 3] : [periodCount >= golay_type*4-2 && periodCount <= golay_type*4+2 && peak == true ]
  BufferFirst -> WaitForNext [order 2]
  (default) -> Reset
  WaitForNext -> WaitForNext [order 4]
  SequentialDetected -> Reset
  CalculateDiff -> SequentialDetected [order 2] : [peakCount >= preambleSequentialDetect]
  data: peak input boolean; periodCount local int32; rst input boolean; preambleSequentialDetect parameter int32; err output boolean; detected output boolean; peakCount local int32; golay_type parameter int32; possible output

== matlab function rev0BB/MATLAB Function ==
  data: symbolIn input; valid input; lineWidth input
function decodeText(symbolIn,valid,lineWidth)
%DECODE_TEXT Decodes text as it is recieved
persistent count;
persistent lineCount;
persistent symbolBuffer;
persistent prevValid;

if isempty(prevValid)
    prevValid = false;
end
    
if isempty(count)
    count = 0;
end

if isempty(symbolBuffer)
    symbolBuffer = 0;
end

if isempty(lineCount)
    lineCount = 0;
end

if(valid)
    %Buffer the newest symbol (binary)
    newBit = 0;
    if(symbolIn ~= 0 )
        newBit = 1;
    end

    symbolBuffer = symbolBuffer * 2;
    symbolBuffer = symbolBuffer + newBit;
    count = count+1;

    %%have full char, now decode and reset
    if(count >= 8)
        if(symbolBuffer <= 2^7)
            newChar = char(symbolBuffer);
        else
            newChar = '$';
        end
        fprintf('%s', newChar);
        count = 0;
        symbolBuffer = 0;
        lineCount = lineCount+1;
        if(lineCount>lineWidth && newChar==' ')
            fprintf('\n');
            lineCount = 0;
        end
    end
%else
%    count = 0;
%    symbolBuffer = 0;
end

== stateflow chart rev0BB/receiver/slim_fast_rx1/preamble_detect ==
  settings: executeAtInitialization=1
  state Lost
    entry:
    err = true;
    periodCount = int32(0);
  state Reset
    entry:
    err=false;
    detected=false;
    periodCount = int32(0);
    peakCount = int32(0);
  state WaitForNext
    entry:
    periodCount = periodCount + int32(1);
  state CalculateDiff
    entry:
    peakCount = peakCount + int32(1);
    periodCount = int32(1);
  state BufferFirst
    entry:
    periodCount = int32(1);
  state SequentialDetected
    entry:
    detected=true;
  CalculateDiff -> Reset [order 1] : [rst == true]
  WaitForNext -> Reset [order 1] : [rst == true]
  WaitForNext -> Lost [order 2] : [periodCount > golay_type*4+4]
  Lost -> Reset
  CalculateDiff -> WaitForNext [order 3]
  BufferFirst -> Reset [order 1] : [rst == true]
  Reset -> BufferFirst : [peak == true]
  WaitForNext -> CalculateDiff [order 3] : [periodCount >= golay_type*4-2 && periodCount <= golay_type*4+2 && peak == true ]
  BufferFirst -> WaitForNext [order 2]
  (default) -> Reset
  WaitForNext -> WaitForNext [order 4]
  SequentialDetected -> Reset
  CalculateDiff -> SequentialDetected [order 2] : [peakCount >= preambleSequentialDetect]
  data: peak input boolean; periodCount local int32; rst input boolean; preambleSequentialDetect parameter int32; err output boolean; detected output boolean; peakCount local int32; golay_type parameter int32

== stateflow chart rev0BB/receiver/slow_rx_baseband_outer/slow_rx_baseband_enabled/slow_rx_baseband/CoarseCFO_est/cfo_est_control ==
  settings: executeAtInitialization=1
  state Reset
    entry:
    buffer = false;
    calcDiff = false;
    periodCount = int32(0);
    peakCount = int32(0);
  state WaitForNext
    entry:
    buffer = false;
    calcDiff = false;
    periodCount = periodCount + int32(1);
  state BufferFirst
    entry:
    buffer = true;
    cur = correlation;
    calcDiff = false;
    periodCount = int32(1);
  state CalculateDiff
    entry:
    buffer = true;
    prev = cur;
    cur = correlation;
    calcDiff = true;
    peakCount = peakCount + int32(1);
    periodCount = int32(1);
  state HoldDiff
    entry:
    buffer = false;
    calcDiff = false;
  CalculateDiff -> Reset [order 1] : [rst == true]
  WaitForNext -> Reset [order 1] : [rst == true]
  CalculateDiff -> WaitForNext [order 3]
  BufferFirst -> Reset [order 1] : [rst == true]
  Reset -> BufferFirst : [peak == true]
  BufferFirst -> WaitForNext [order 3]
  WaitForNext -> CalculateDiff [order 3] : [periodCount >= golay_type ]
  (default) -> Reset
  WaitForNext -> WaitForNext [order 4]
  WaitForNext -> HoldDiff [order 2] : [stp == true]
  HoldDiff -> Reset : [rst == true]
  BufferFirst -> HoldDiff [order 2] : [stp == true]
  CalculateDiff -> HoldDiff [order 2] : [stp == true]
  data: peak input boolean; cur output; prev output; calcDiff output boolean; periodCount local int32; correlation input; stp input boolean; rst input boolean; peakCount output int32; buffer output boolean; golay_type parameter int32

== stateflow chart rev0BB/receiver/slim_fast_rx2/preamble_detect ==
  settings: executeAtInitialization=1
  state Lost
    entry:
    err = true;
    periodCount = int32(0);
  state Reset
    entry:
    err=false;
    detected=false;
    periodCount = int32(0);
    peakCount = int32(0);
  state WaitForNext
    entry:
    periodCount = periodCount + int32(1);
  state CalculateDiff
    entry:
    peakCount = peakCount + int32(1);
    periodCount = int32(1);
  state BufferFirst
    entry:
    periodCount = int32(1);
  state SequentialDetected
    entry:
    detected=true;
  CalculateDiff -> Reset [order 1] : [rst == true]
  WaitForNext -> Reset [order 1] : [rst == true]
  WaitForNext -> Lost [order 2] : [periodCount > golay_type*4+4]
  Lost -> Reset
  CalculateDiff -> WaitForNext [order 3]
  BufferFirst -> Reset [order 1] : [rst == true]
  Reset -> BufferFirst : [peak == true]
  WaitForNext -> CalculateDiff [order 3] : [periodCount >= golay_type*4-2 && periodCount <= golay_type*4+2 && peak == true ]
  BufferFirst -> WaitForNext [order 2]
  (default) -> Reset
  WaitForNext -> WaitForNext [order 4]
  SequentialDetected -> Reset
  CalculateDiff -> SequentialDetected [order 2] : [peakCount >= preambleSequentialDetect]
  data: peak input boolean; periodCount local int32; rst input boolean; preambleSequentialDetect parameter int32; err output boolean; detected output boolean; peakCount local int32; golay_type parameter int32

== stateflow chart rev0BB/receiver/slow_rx_baseband_outer/slow_rx_baseband_enabled/slow_rx_baseband/preamble_data_ctrl/cef_eq_fsm ==
  settings: executeAtInitialization=1
  state Error
    entry:
    err = true;
    waiting = false;
  state Waiting
    entry:
    stf = false;
    cef = false;
    cef_early = false;
    data = false;
    err = false;
    ack = false;
    ack_done = false;
    ack_trigger = false;
    ack_count = uint8(0);
    ack_dst = uint8(0);
    waiting = true;
    stfCount = int32(0);
    stfPeaks = int32(0);
    cefCount = int32(0);
    cefSymb=int16(0);
  state STFFirst
    entry:
    stf = true;
    cef = false;
    cef_early = false;
    data = false;
    err = false;
    ack = false;
    ack_done = false;
    waiting = false;
    stfCount = 1;
    stfPeaks = stfPeaks + 1;
    cefSymb=int16(0);
  state STF
    entry:
    stf = true;
    cef = false;
    cef_early = false;
    data = false;
    err = false;
    ack = false;
    ack_done = false;
    waiting = false;
    stfCount = stfCount+1;
    cefSymb=int16(0);
  state CEF_Early_Warning
    entry:
    stf = false;
    cef = true;
    cef_early = true;
    data = false;
    err = false;
    waiting = false;
    ack = false;
    ack_done = false;
    cefSymb = cefGen(cefCount+1);
    cefCount = cefCount +1;
  state LastSym
    entry:
    stf = false;
    cef = false;
    cef_early = false;
    data = true;
    err = false;
    waiting = false;
    ack = false;
    ack_done = false;
    cefSymb=int16(0);
  state CEF_Decision
    entry:
    stf = false;
    cef = true;
    cef_early = false;
    data = false;
    err = false;
    waiting = false;
    ack = false;
    ack_done = false;
    cefSymb = cefGen(cefCount+1);
    cefCount = cefCount +1;
  state CEF
    entry:
    stf = false;
    cef = true;
    cef_early = false;
    data = false;
    err = false;
    waiting = false;
    ack = false;
    ack_done = false;
    cefSymb = cefGen(cefCount+1);
    cefCount = cefCount +1;
  state Ack_First
    entry:
    stf = false;
    cef = true;
    cef_early = false;
    data = false;
    err = false;
    waiting = false;
    ack = true;
    ack_done = false;
    cefSymb = int16(0);
    cefCount = int32(1);
  state Ack_Done
    entry:
    stf = false;
    cef = false;
    cef_early = false;
    data = false;
    err = false;
    waiting = false;
    ack = true;
    ack_done = true;
    ack_trigger = false;
    cefSymb = int16(0);
    cefCount = int32(0);
  state Ack_Wait
    entry:
    stf = false;
    cef = true;
    cef_early = false;
    data = false;
    err = false;
    waiting = false;
    ack = true;
    ack_done = false;
    ack_trigger = false;
    cefSymb = int16(0);
    cefCount = cefCount +1;
  state Ack_Ca
    entry:
    stf = false;
    cef = true;
    cef_early = false;
    data = false;
    err = false;
    waiting = false;
    ack = true;
    ack_done = false;
    ack_trigger = true;
    ack_dst =  bitsrl(ack_dst, 1);
    cefSymb = int16(0);
    cefCount = int32(1);
    ack_count = ack_count + uint8(1);
  state Ack_Cb
    entry:
    stf = false;
    cef = true;
    cef_early = false;
    data = false;
    err = false;
    waiting = false;
    ack = true;
    ack_done = false;
    ack_trigger = true;
    ack_dst =  bitor(bitsrl(ack_dst, 1), bitsll(1, 7));
    cefSymb = int16(0);
    cefCount = int32(1);
    ack_count = ack_count + uint8(1);
  CEF_Decision -> Error [order 1] : [cefCount >= golay_type && ((stf_start == true && cef_start == true) || (stf_start == false && cef_start == false))]
  Ack_Wait -> Error [order 1] : [cefCount >= golay_type && ((stf_start == true && cef_start == true) || (stf_start == false && cef_start == false))]
  STF -> Error [order 1] : [stfCount >= golay_type && (stf_start==false && cef_start == false) || (stf_start==true && cef_start == true) || (cef_start == true && (stfPeaks < minSTFPeaks || stfPeaks > (x_STFRepCount+1)))]
  Error -> Waiting
  (default) -> Waiting
  CEF_Early_Warning -> CEF_Early_Warning [order 2]
  CEF -> CEF [order 2]
  CEF_Decision -> CEF_Decision [order 4]
  STFFirst -> STF
  Waiting -> STFFirst : [stf_start==true]
  STF -> CEF_Decision [order 2] : [stfCount >= golay_type && cef_start == true && stfPeaks >= minSTFPeaks && stfPeaks <= (x_STFRepCount+1) ]
  CEF_Decision -> CEF [order 3] : [cefCount >= golay_type && stf_start == true]
  STF -> STFFirst [order 3] : [stfCount >= golay_type && stf_start==true]
  STF -> STF [order 4]
  LastSym -> Waiting
  CEF_Early_Warning -> LastSym [order 1] : [cefCount >= cefLen]
  CEF -> CEF_Early_Warning [order 1] : [cefCount >= cefLen-cefEarlyWarning]
  CEF_Decision -> Ack_First [order 2] : [cefCount >= golay_type && cef_start == true]
  Ack_Done -> Waiting
  Ack_First -> Ack_Wait
  Ack_Wait -> Ack_Wait [order 4]
  Ack_Wait -> Ack_Cb [order 2] : [cefCount >= golay_type && stf_start == true]
  Ack_Wait -> Ack_Ca [order 3] : [cefCount >= golay_type && cef_start == true]
  Ack_Ca -> Ack_Done [order 2] : [ack_count >= 8]
  Ack_Cb -> Ack_Done [order 2] : [ack_count >= 8]
  Ack_Cb -> Ack_Wait [order 1] : [ack_count < 8]
  Ack_Ca -> Ack_Wait [order 1] : [ack_count < 8]
  data: ind function_input; symb function_output boolean; stf_start input boolean; cef_start input boolean; data output boolean; err output boolean; cefSymb output int16; stf output boolean; cef output boolean; cefCount output int32; stfCount local int32; stfLen parameter int32; cefLen parameter int32; cefEarlyWarning parameter int32; cef_early output boolean; waiting output boolean; golay_type parameter; ack_done output boolean; ack output boolean; ack_dst output uint8; ack_count output uint8; ack_trigger output boolean; x_STFRepCount parameter; minSTFPeaks parameter; stfPeaks local
  function symb = cefGen(ind):
    | function symb = cefGen(ind)
    | %128
    | % Ga_128 = [+1, +1, -1, -1, -1, -1, -1, -1, -1, +1, -1, +1, +1, -1, -1, +1, +1, +1, -1, -1, +1, +1, +1, +1, -1, +1, -1, +1, -1, +1, +1, -1, -1, -1, +1, +1, +1, +1, +1, +1, +1, -1, +1, -1, -1, +1, +1, -1, +1, +1, -1, -1, +1, +1, +1, +1, -1, +1, -1, +1, -1, +1, +1, -1, +1, +1, -1, -1, -1, -1, -1, -1, -1, +1, -1, +1, +1, -1, -1, +1, +1, +1, -1, -1, +1, +1, +1, +1, -1, +1, -1, +1, -1, +1, +1, -1, +1, +1, -1, -1, -1, -1, -1, -1, -1, +1, -1, +1, +1, -1, -1, +1, -1, -1, +1, +1, -1, -1, -1, -1, +1, -1, +1, -1, +1, -1, -1, +1];
    | % Gb_128 = [-1, -1, +1, +1, +1, +1, +1, +1, +1, -1, +1, -1, -1, +1, +1, -1, -1, -1, +1, +1, -1, -1, -1, -1, +1, -1, +1, -1, +1, -1, -1, +1, +1, +1, -1, -1, -1, -1, -1, -1, -1, +1, -1, +1, +1, -1, -1, +1, -1, -1, +1, +1, -1, -1, -1, -1, +1, -1, +1, -1, +1, -1, -1, +1, +1, +1, -1, -1, -1, -1, -1, -1, -1, +1, -1, +1, +1, -1, -1, +1, +1, +1, -1, -1, +1, +1, +1, +1, -1, +1, -1, +1, -1, +1, +1, -1, +1, +1, -1, -1, -1, -1, -1, -1, -1, +1, -1, +1, +1, -1, -1, +1, -1, -1, +1, +1, -1, -1, -1, -1, +1, -1, +1, -1, +1, -1, -1, +1];
    | % 
    | % Gu_512 = cat(2, -Gb_128, -Ga_128, Gb_128, -Ga_128);
    | % Gv_512 = cat(2, -Gb_128, Ga_128, -Gb_128, -Ga_128);
    | % Gv_128 = Gv_512(1:1:128);
    | 
    | % xSpectrum_CEF = cat(2, Gu_512, Gv_512, Gu_512, Gv_512, Gu_512, Gv_512, Gu_512, Gv_512, Gu_512, Gv_512, Gv_128);
    | % xSpectrum_CEF = cat(2, Gu_512, Gv_512, Gv_512);
    | 
    | %32
    | Ga_32  = [+1, +1, +1, +1, +1, -1, +1, -1, -1, -1, +1, +1, +1, -1, -1, +1, +1, +1, -1, -1, +1, -1, -1, +1, -1, -1, -1, -1, +1, -1, +1, -1];
    | Gb_32  = [-1, -1, -1, -1, -1, +1, -1, +1, +1, +1, -1, -1, -1, +1, +1, -1, +1, +1, -1, -1, +1, -1, -1, +1, -1, -1, -1, -1, +1, -1, +1, -1];
    | 
    | Gu_128_s = cat(2, -Gb_32, -Ga_32, Gb_32, -Ga_32);
    | Gv_128_s = cat(2, -Gb_32, Ga_32, -Gb_32, -Ga_32);
    | 
    | xSpectrum_CEF_short = cat(2, Gu_128_s, Gv_128_s, Gu_128_s, Gv_128_s, Gu_128_s, Gv_128_s, Gu_128_s, Gv_128_s, Gu_128_s, Gv_128_s, Gu_128_s, Gv_128_s, Gu_128_s, Gv_128_s);
    | %xSpectrum_CEF_short = cat(2, Gu_128_s, Gv_128_s, Gu_128_s, Gv_128_s, Gu_128_s, Gv_128_s, Gu_128_s, Gv_128_s, Gu_128_s, Gv_128_s, Gu_128_s, Gv_128_s, Gu_128_s, Gv_128_s, Gu_128_s, Gv_128_s, Gu_128_s, Gv_128_s);
    | %xSpectrum_CEF_short = cat(2, Gu_128_s, Gv_128_s, Gu_128_s, Gv_128_s, Gu_128_s, Gv_128_s, Gu_128_s, Gv_128_s, Gu_128_s, Gv_128_s, Gu_128_s, Gv_128_s, Gu_128_s, Gv_128_s, Gu_128_s, Gv_128_s, Gu_128_s, Gv_128_s, Gu_128_s, Gv_128_s, Gu_128_s, Gv_128_s, Gu_128_s, Gv_128_s, Gu_128_s, Gv_128_s, Gu_128_s, Gv_128_s);
    | 
    | 
    | symb = int16(xSpectrum_CEF_short(ind));
    | 
    | end

== stateflow chart rev0BB/receiver/slow_rx_baseband_outer/slow_rx_baseband_enabled/slow_rx_baseband/preamble_data_ctrl/data_control ==
  settings: executeAtInitialization=1
  state Data
    entry:
    valid = true;
    last = false;
    dataCount = dataCount + int32(1);
  state LastSym
    entry:
    valid = true;
    last = true;
    dataCount = dataCount + int32(1);
  state Waiting
    entry:
    valid = false;
    last = false;
    startCount = int32(0);
    dataCount = int32(0);
    waitCount = int32(0);
  Data -> Data [order 2]
  (default) -> Waiting
  Waiting -> Data : [preamble_done == true]
  LastSym -> Waiting
  Data -> LastSym [order 1] : [dataCount >= dataLenSymbols-1]
  data: preamble_done input boolean; valid output boolean; startCount local int32; dataCount local int32; buffer local boolean size=8; guardInt parameter int32; guardTol parameter int32; waitCount local int32; wordLen parameter int32; dataLenSymbols parameter int32; last output boolean
